simulink library "astroDynamics"  (R2015b)
settings: Solver=VariableStepAuto  StartTime=0.0  StopTime=10.0  RelTol=1e-3
settings Model: Creator=yyas16  LastModifiedBy=yyas16

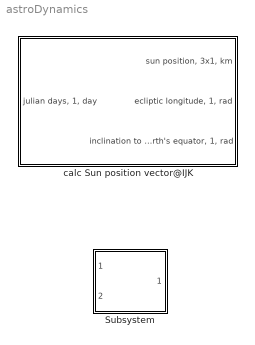
== system astroDynamics ==
  Subsystem : Subsystem
  calc Sun position vector@IJK : Subsystem

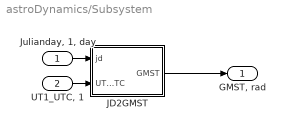
== system astroDynamics/Subsystem ==
  "Julianday, 1, day" : Inport
  "UT1_UTC, 1" : Inport  Port=2
  JD2GMST : MATLAB Function  TreatAsAtomicUnit=on
  "GMST, rad" : Outport
  wires:
  JD2GMST/1(GMST) -> "GMST, rad"/1
  "Julianday, 1, day"/1 -> JD2GMST/1(jd)
  "UT1_UTC, 1"/1 -> JD2GMST/2(UT1_UTC)

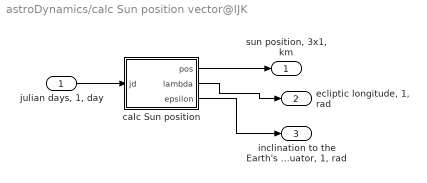
== system astroDynamics/calc Sun position vector@IJK ==
  "julian days, 1, day" : Inport
  calc Sun position : MATLAB Function  TreatAsAtomicUnit=on
  "sun position, 3x1, km" : Outport
  "ecliptic longitude, 1, rad" : Outport  Port=2
  "inclination to the Earth's equator, 1, rad" : Outport  Port=3
  wires:
  "julian days, 1, day"/1 -> calc Sun position/1(jd)
  calc Sun position/1(pos) -> "sun position, 3x1, km"/1
  calc Sun position/2(lambda) -> "ecliptic longitude, 1, rad"/1
  calc Sun position/3(epsilon) -> "inclination to the Earth's equator, 1, rad"/1

== matlab function astroDynamics/calc Sun position vector@IJK/calc Sun position ==
  data: jd input; pos output; lambda output; epsilon output
function [pos, lambda, epsilon] = calcSunPos(jd)
%#codegen
% cf.	Montenbruck, O., and Gill, E., Satellite Orbits,
% Berlin, Heidelberg: Springer Science & Business Media, 2012.
%
% in , jd: julian days, 1, [day]
% out, pos:   sun postiion @IJK, 3x1, [km]
%      lambda: ecliptic longitude, 1, [rad]
%      epsilon: inclination of the cliptic relative to the Earth's equator,
%      [rad]

DEG2RAD = pi / 180.0;

T   = (jd - 2451545.0) / 36525.0; % Julian century
M   = (357.5291092 + 35999.05034 * T) * DEG2RAD; % mean anomaly of the Sun, [rad]
lam = M + ...
    282.9400 * DEG2RAD...
    + (6892.0 * sin(M) / 3600.0 + 72.0 * sin(M) / 3600.0) * DEG2RAD; % ecliptic longitude [rad]
beta = 0.0; % ecliptic latitude [rad] %

r = (149.619 - 2.499 * cos(M) - 0.021 * cos(2.0 * M)) * 10^6; % distance[km];

epsilon = 23.43929111 / 180.0 * pi;

pos = [r * cos(lam)
    r * sin(lam) * cos(epsilon)
    r * sin(lam) * sin(epsilon)];
lambda= lam;

== matlab function astroDynamics/Subsystem/JD2GMST ==
  data: jd input; GMST output; UT1_UTC input
function GMST = fcn(jd, UT1_UTC)
%#codegen

MJD = jd - 2400000.5 + UT1_UTC / 86400.0;
ut1_ss = (MJD - floor(MJD)) * 86400.0;
MJD = floor(MJD);

T = (MJD - 51544.5) / 36525.0;

GMST = 8640184.812866 * T;

GMST = GMST + (-6.2e-6 * T + 0.093104) * T * T + 24110.54841;

dsdmr = 1.002737909350795 + 5.9006e-11 * T -5.9e-15 * T * T;

GMST = GMST + dsdmr * ut1_ss;

GMST = GMST - 86400.0 * floor(GMST / 86400.0);
